simulink model "cc_motor_otimization"  (R2019a)
settings: Solver=VariableStepAuto  StartTime=0.0  StopTime=10  RelTol=1e-3
settings Model: Creator=bren0  LastModifiedBy=bren0

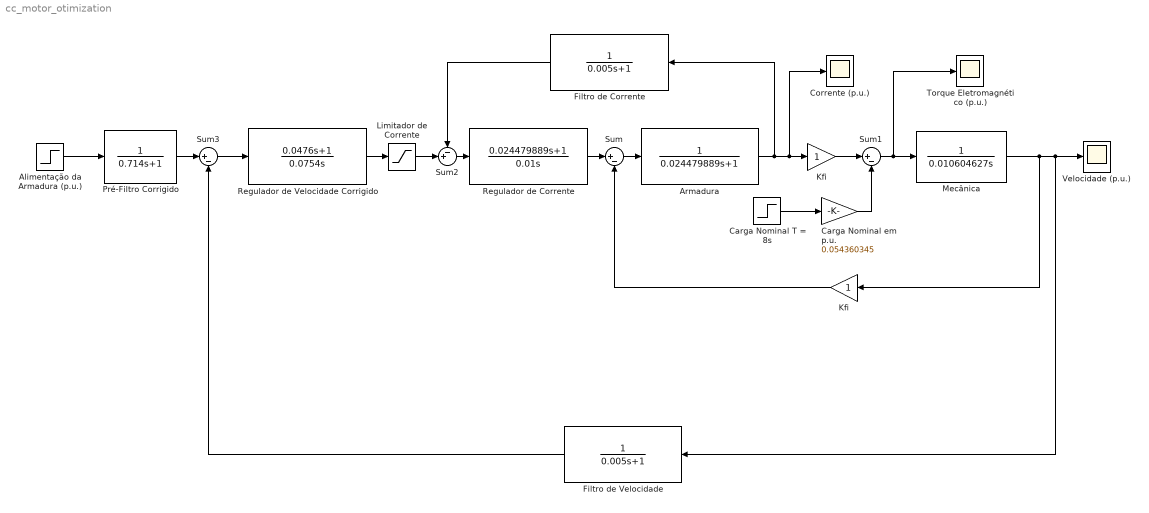
== system cc_motor_otimization ==
  " Kfi" : Gain
  Alimentação da Armadura (p.u.) : Step  Time=0  SampleTime=0.001
  Armadura : TransferFcn  Denominator=[0.024479889, 1]
  Carga Nominal em p.u. : Gain  Gain=0.054360345
  Carga Nominal T = 8s : Step  Time=8  SampleTime=0.001
  Corrente (p.u.) : Scope
  Filtro de Corrente : TransferFcn  Denominator=[0.005, 1]
  Filtro de Velocidade : TransferFcn  Denominator=[0.005, 1]
  Kfi : Gain
  Limitador de Corrente : Saturate  UpperLimit=0.271801726
  Mecânica : TransferFcn  Denominator=[0.010604627, 0]
  Pré-Filtro Corrigido : TransferFcn  Denominator=[0.714, 1]
  Regulador de Corrente : TransferFcn  Numerator=[0.024479889 1]  Denominator=[0.01, 0]
  Regulador de Velocidade Corrigido : TransferFcn  Numerator=[0.0476, 1]  Denominator=[0.0754, 0]
  Sum : Sum  Inputs=|+-
  Sum1 : Sum  Inputs=|+-
  Sum2 : Sum  Inputs=-+|
  Sum3 : Sum  Inputs=|+-
  Torque Eletromagnético (p.u.) : Scope
  Velocidade (p.u.) : Scope
  wires:
  Sum/1 -> Armadura/1
  Armadura/1 -> Filtro de Corrente/1, Kfi/1, Corrente (p.u.)/1
  Kfi/1 -> Sum1/1
  Sum1/1 -> Torque Eletromagnético (p.u.)/1, Mecânica/1
  " Kfi"/1 -> Sum/2
  Carga Nominal T = 8s/1 -> Carga Nominal em p.u./1
  Carga Nominal em p.u./1 -> Sum1/2
  Regulador de Corrente/1 -> Sum/1
  Sum2/1 -> Regulador de Corrente/1
  Filtro de Corrente/1 -> Sum2/1
  Sum3/1 -> Regulador de Velocidade Corrigido/1
  Filtro de Velocidade/1 -> Sum3/2
  Mecânica/1 -> Filtro de Velocidade/1, Velocidade (p.u.)/1, " Kfi"/1
  Alimentação da Armadura (p.u.)/1 -> Pré-Filtro Corrigido/1
  Pré-Filtro Corrigido/1 -> Sum3/1
  Limitador de Corrente/1 -> Sum2/2
  Regulador de Velocidade Corrigido/1 -> Limitador de Corrente/1
